simulink library "halin"  (R2021b)
settings: Solver=VariableStepAuto  StartTime=0.0  StopTime=10.0  RelTol=1e-3
undefined symbols (not defined in the file): KHAL_CAN1ABM1E2E_flg, KHAL_CAN1ESC1E2E_flg, KHAL_CAN1ESC5E2E_flg, KHAL_CAN1ESC7E2E_flg, KHAL_CAN1FCM2E2E_flg, KHAL_CAN1FCM3E2E_flg, KHAL_CAN1FCM4E2E_flg, KHAL_CAN3BMS1E2E_flg, KHAL_CAN3BMS6E2E_flg, KHAL_CAN3CCU1E2E_flg, KHAL_CAN3CCU2E2E_flg, KHAL_CAN3MCUF1E2E_flg, KHAL_CAN3MCUR1E2E_flg, KHAL_CAN3Shifter1E2E_flg, TRUE
libraries: simulink x420, FVT_lib x149, hcu_lib x49
(part 6 of 14)

== system halin/HAL_IN/CAN1/FCM3 ==
  DT_CAN1_SG_FCM3 : Inport
  0x82 : Constant  Value=0x82
  0xa0 : Constant  Value=0xa0
  ACCObjDist : Subsystem
  ACCObjRelSpd : Subsystem
  ADASForceIdle : Subsystem
  BitwiseAND{,1..9} (10 alike) : simulink/Logic and Bit Operations/Bitwise Operator  logicop=AND  UseBitMask=on  BitMask=0xFF  BitMaskRealWorld=Stored Integer
  BitwiseOR{,2,4..5} (4 alike) : simulink/Logic and Bit Operations/Bitwise Operator  logicop=OR  UseBitMask=off  BitMask=bin2dec('11011001')  BitMaskRealWorld=Stored Integer
  BitwiseOR1 : simulink/Logic and Bit Operations/Bitwise Operator  logicop=OR  UseBitMask=off  NumInputPorts=3  BitMask=bin2dec('11011001')  BitMaskRealWorld=Stored Integer
  BitwiseOR3 : simulink/Logic and Bit Operations/Bitwise Operator  logicop=OR  UseBitMask=off  NumInputPorts=3  BitMask=bin2dec('11011001')  BitMaskRealWorld=Stored Integer
  DDM_CS&RC_Comparison : FVT_lib/hal/DDM_CS&RC_Comparison  MsgCycleTime=10
  Data Type Conversion{,1..9} (10 alike) : DataTypeConversion  OutDataTypeStr=uint8
  FCM3Checksum : Subsystem
  FCM3LifeCount : Subsystem
  KHAL_CAN1FCM3E2E_flg : Constant  Value=KHAL_CAN1FCM3E2E_flg
  LeftShift : ArithShift  BitShiftNumber=3  BitShiftDirection=Left
  LeftShift1 : ArithShift  BitShiftNumber=3  BitShiftDirection=Left
  LeftShift2 : ArithShift  BitShiftNumber=6  BitShiftDirection=Left
  LeftShift3 : ArithShift  BitShiftDirection=Left
  LeftShift4 : ArithShift  BitShiftDirection=Left
  LeftShift5 : ArithShift  BitShiftNumber=4  BitShiftDirection=Left
  MessageRollingCounter : FVT_lib/hal/MessageRollingCounter  CounterMAX=14  task_time_ms=5  msg_time_ms=10
  Mux : Mux  Inputs=7
  RightShift : ArithShift  BitShiftNumber=8
  RightShift1 : ArithShift
  RightShift2 : ArithShift  BitShiftNumber=8
  RightShift3 : ArithShift
  bus_selector : BusSelector  OutputSignals=CAN1_ACC_ObjDist,CAN1_ACC_ObjRelSpd,CAN1_ADAS_ForceIdle,CAN1_ADAS_ShftPosnReq,CAN1_ADAS_ShftPosnReq_A,CAN1_ADAS_VehSpdLim,CAN1_FCM3_Checksum,CAN1_FCM3_LifeCount
  bus_selector1 : BusSelector  OutputSignals=CAN1_ACC_ObjDist
  bus_selector2 : BusSelector  OutputSignals=CAN1_ACC_ObjRelSpd
  bus_selector3 : BusSelector  OutputSignals=CAN1_ADAS_ForceIdle
  bus_selector4 : BusSelector  OutputSignals=CAN1_FCM3_Checksum
  bus_selector5 : BusSelector  OutputSignals=CAN1_FCM3_LifeCount
  constant : Constant  Value=0x0  OutDataTypeStr=uint8
  constant1 : Constant  Value=0x0  OutDataTypeStr=uint8
  VHAL_FCM3CSErr_flg : Outport
  VHAL_FCM3RCErr_flg : Outport  Port=2
  VHAL_ACCObjDist_m : Outport  Port=3
  VHAL_ACCObjRelSpd_mps : Outport  Port=4
  VHAL_ADASForceIdle_flg : Outport  Port=5
  VHAL_FCM3Checksum_enum : Outport  Port=6
  VHAL_FCM3LifeCount_enum : Outport  Port=7
  wires:
  DT_CAN1_SG_FCM3/1 -> [DT_CAN1_SG_FCM3]
  [DT_CAN1_SG_FCM3] -> bus_selector/1
  bus_selector/1 -> [CAN1_ACC_ObjDist]  "<CAN1_ACC_ObjDist>"
  [CAN1_ACC_ObjDist] -> RightShift/1, RightShift1/1
  RightShift/1 -> BitwiseAND/1
  BitwiseAND/1 -> [Byte_3_CAN1_ACC_ObjDist]
  RightShift1/1 -> BitwiseAND1/1
  BitwiseAND1/1 -> [Byte_4_CAN1_ACC_ObjDist]
  bus_selector/2 -> [CAN1_ACC_ObjRelSpd]  "<CAN1_ACC_ObjRelSpd>"
  [CAN1_ACC_ObjRelSpd] -> RightShift2/1, RightShift3/1
  RightShift2/1 -> BitwiseAND2/1
  BitwiseAND2/1 -> [Byte_5_CAN1_ACC_ObjRelSpd]
  RightShift3/1 -> BitwiseAND3/1
  BitwiseAND3/1 -> [Byte_6_CAN1_ACC_ObjRelSpd]
  bus_selector/3 -> [CAN1_ADAS_ForceIdle]  "<CAN1_ADAS_ForceIdle>"
  [CAN1_ADAS_ForceIdle] -> LeftShift/1
  LeftShift/1 -> BitwiseAND4/1
  BitwiseAND4/1 -> [Byte_5_CAN1_ADAS_ForceIdle]
  bus_selector/4 -> [CAN1_ADAS_ShftPosnReq]  "<CAN1_ADAS_ShftPosnReq>"
  [CAN1_ADAS_ShftPosnReq] -> LeftShift1/1
  LeftShift1/1 -> BitwiseAND5/1
  BitwiseAND5/1 -> [Byte_3_CAN1_ADAS_ShftPosnReq]
  bus_selector/5 -> [CAN1_ADAS_ShftPosnReq_A]  "<CAN1_ADAS_ShftPosnReq_A>"
  [CAN1_ADAS_ShftPosnReq_A] -> LeftShift2/1
  LeftShift2/1 -> BitwiseAND6/1
  BitwiseAND6/1 -> [Byte_3_CAN1_ADAS_ShftPosnReq_A]
  bus_selector/6 -> [CAN1_ADAS_VehSpdLim]  "<CAN1_ADAS_VehSpdLim>"
  [CAN1_ADAS_VehSpdLim] -> LeftShift3/1
  LeftShift3/1 -> BitwiseAND7/1
  BitwiseAND7/1 -> [Byte_0_CAN1_ADAS_VehSpdLim]
  bus_selector/7 -> [CAN1_FCM3_Checksum]  "<CAN1_FCM3_Checksum>"
  [CAN1_FCM3_Checksum] -> LeftShift4/1
  LeftShift4/1 -> BitwiseAND8/1
  BitwiseAND8/1 -> [Byte_7_CAN1_FCM3_Checksum]
  bus_selector/8 -> [CAN1_FCM3_LifeCount]  "<CAN1_FCM3_LifeCount>"
  [CAN1_FCM3_LifeCount] -> LeftShift5/1
  LeftShift5/1 -> BitwiseAND9/1
  BitwiseAND9/1 -> [Byte_5_CAN1_FCM3_LifeCount]
  Data Type Conversion/1 -> BitwiseOR/1
  [Byte_0_CAN1_ADAS_VehSpdLim] -> Data Type Conversion/1
  BitwiseOR/1 -> [Byte_0]
  constant/1 -> [Byte_1]
  constant1/1 -> [Byte_2]
  Data Type Conversion1/1 -> BitwiseOR1/1
  [Byte_3_CAN1_ACC_ObjDist] -> Data Type Conversion1/1
  Data Type Conversion2/1 -> BitwiseOR1/2
  [Byte_3_CAN1_ADAS_ShftPosnReq] -> Data Type Conversion2/1
  Data Type Conversion3/1 -> BitwiseOR1/3
  [Byte_3_CAN1_ADAS_ShftPosnReq_A] -> Data Type Conversion3/1
  BitwiseOR1/1 -> [Byte_3]
  Data Type Conversion4/1 -> BitwiseOR2/1
  [Byte_4_CAN1_ACC_ObjDist] -> Data Type Conversion4/1
  BitwiseOR2/1 -> [Byte_4]
  Data Type Conversion5/1 -> BitwiseOR3/1
  [Byte_5_CAN1_ACC_ObjRelSpd] -> Data Type Conversion5/1
  Data Type Conversion6/1 -> BitwiseOR3/2
  [Byte_5_CAN1_ADAS_ForceIdle] -> Data Type Conversion6/1
  Data Type Conversion7/1 -> BitwiseOR3/3
  [Byte_5_CAN1_FCM3_LifeCount] -> Data Type Conversion7/1
  BitwiseOR3/1 -> [Byte_5]
  Data Type Conversion8/1 -> BitwiseOR4/1
  [Byte_6_CAN1_ACC_ObjRelSpd] -> Data Type Conversion8/1
  BitwiseOR4/1 -> [Byte_6]
  Data Type Conversion9/1 -> BitwiseOR5/1
  [Byte_7_CAN1_FCM3_Checksum] -> Data Type Conversion9/1
  BitwiseOR5/1 -> [Byte_7]
  [Byte_0] -> Mux/1
  [Byte_1] -> Mux/2
  [Byte_2] -> Mux/3
  [Byte_3] -> Mux/4
  [Byte_4] -> Mux/5
  [Byte_5] -> Mux/6
  [Byte_6] -> Mux/7
  Mux/1 -> [VHAL_CAN1FCM3noCS_raw]
  KHAL_CAN1FCM3E2E_flg/1 -> DDM_CS&RC_Comparison/1
  0xa0/1 -> DDM_CS&RC_Comparison/2
  0x82/1 -> DDM_CS&RC_Comparison/3
  [VHAL_CAN1FCM3noCS_raw] -> DDM_CS&RC_Comparison/4
  [Byte_7] -> DDM_CS&RC_Comparison/5
  [RC_ECU] -> DDM_CS&RC_Comparison/6
  MessageRollingCounter/1 -> DDM_CS&RC_Comparison/7
  DDM_CS&RC_Comparison/1 -> VHAL_FCM3CSErr_flg/1
  DDM_CS&RC_Comparison/2 -> VHAL_FCM3RCErr_flg/1
  [DT_CAN1_SG_FCM3] -> bus_selector1/1
  bus_selector1/1 -> ACCObjDist/1(ACC_ObjDist)  "<CAN1_ACC_ObjDist>"
  ACCObjDist/1(VHAL_ACCObjDist_m) -> VHAL_ACCObjDist_m/1
  [DT_CAN1_SG_FCM3] -> bus_selector2/1
  bus_selector2/1 -> ACCObjRelSpd/1(ACC_ObjRelSpd)  "<CAN1_ACC_ObjRelSpd>"
  ACCObjRelSpd/1(VHAL_ACCObjRelSpd_mps) -> VHAL_ACCObjRelSpd_mps/1
  [DT_CAN1_SG_FCM3] -> bus_selector3/1
  bus_selector3/1 -> ADASForceIdle/1(ADAS_ForceIdle)  "<CAN1_ADAS_ForceIdle>"
  ADASForceIdle/1(VHAL_ADASForceIdle_flg) -> VHAL_ADASForceIdle_flg/1
  [DT_CAN1_SG_FCM3] -> bus_selector4/1
  bus_selector4/1 -> FCM3Checksum/1(FCM3_Checksum)  "<CAN1_FCM3_Checksum>"
  FCM3Checksum/1(VHAL_FCM3Checksum_enum) -> VHAL_FCM3Checksum_enum/1
  [DT_CAN1_SG_FCM3] -> bus_selector5/1
  bus_selector5/1 -> FCM3LifeCount/1(FCM3_LifeCount)  "<CAN1_FCM3_LifeCount>"
  FCM3LifeCount/1(VHAL_FCM3LifeCount_enum) -> VHAL_FCM3LifeCount_enum/1, [RC_ECU]

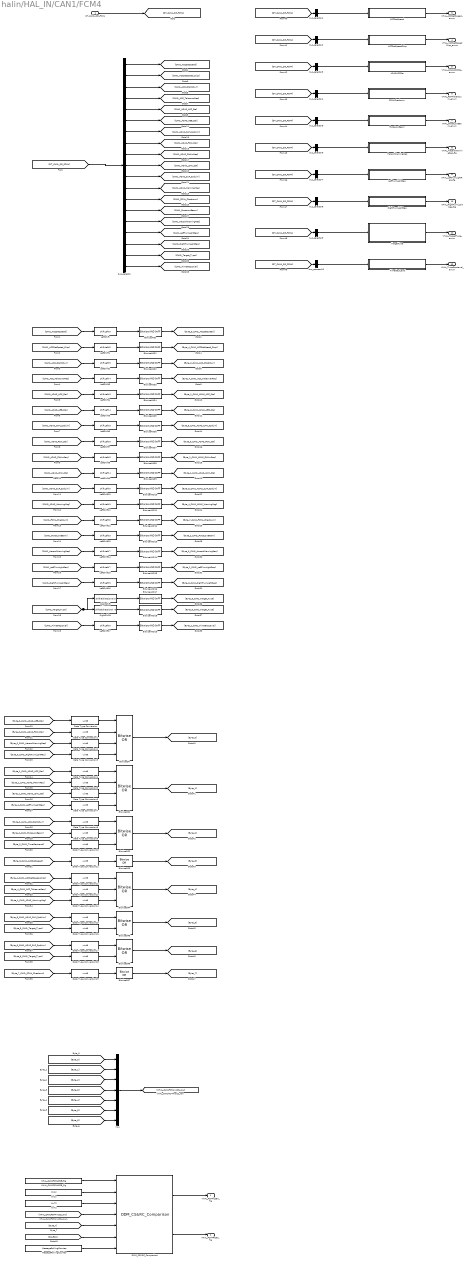
== system halin/HAL_IN/CAN1/FCM4 ==
  DT_CAN1_SG_FCM4 : Inport
  0x1c : Constant  Value=0x1c
  0x72 : Constant  Value=0x72
  ACCSetSpeed : Subsystem
  ACCSetSpeedDisp : Subsystem
  ADASACCSta : Subsystem
  BitwiseAND{,1..19} (20 alike) : simulink/Logic and Bit Operations/Bitwise Operator  logicop=AND  UseBitMask=on  BitMask=0xFF  BitMaskRealWorld=Stored Integer
  BitwiseOR : simulink/Logic and Bit Operations/Bitwise Operator  logicop=OR  UseBitMask=off  NumInputPorts=4  BitMask=bin2dec('11011001')  BitMaskRealWorld=Stored Integer
  BitwiseOR1 : simulink/Logic and Bit Operations/Bitwise Operator  logicop=OR  UseBitMask=off  NumInputPorts=4  BitMask=bin2dec('11011001')  BitMaskRealWorld=Stored Integer
  BitwiseOR2 : simulink/Logic and Bit Operations/Bitwise Operator  logicop=OR  UseBitMask=off  NumInputPorts=3  BitMask=bin2dec('11011001')  BitMaskRealWorld=Stored Integer
  BitwiseOR3 : simulink/Logic and Bit Operations/Bitwise Operator  logicop=OR  UseBitMask=off  BitMask=bin2dec('11011001')  BitMaskRealWorld=Stored Integer
  BitwiseOR4 : simulink/Logic and Bit Operations/Bitwise Operator  logicop=OR  UseBitMask=off  NumInputPorts=3  BitMask=bin2dec('11011001')  BitMaskRealWorld=Stored Integer
  BitwiseOR5 : simulink/Logic and Bit Operations/Bitwise Operator  logicop=OR  UseBitMask=off  NumInputPorts=2  BitMask=bin2dec('11011001')  BitMaskRealWorld=Stored Integer
  BitwiseOR6 : simulink/Logic and Bit Operations/Bitwise Operator  logicop=OR  UseBitMask=off  NumInputPorts=2  BitMask=bin2dec('11011001')  BitMaskRealWorld=Stored Integer
  BitwiseOR7 : simulink/Logic and Bit Operations/Bitwise Operator  logicop=OR  UseBitMask=off  BitMask=bin2dec('11011001')  BitMaskRealWorld=Stored Integer
  DDM_CS&RC_Comparison : FVT_lib/hal/DDM_CS&RC_Comparison  MsgCycleTime=100
  Data Type Conversion{,1..19} (20 alike) : DataTypeConversion  OutDataTypeStr=uint8
  FCM4Checksum : Subsystem
  ForceLowBeam : Subsystem
  HazardWarningReq : Subsystem
  KHAL_CAN1FCM4E2E_flg : Constant  Value=KHAL_CAN1FCM4E2E_flg
  LeftShift{,4,7,10..12,17} (7 alike) : ArithShift  BitShiftDirection=Left
  LeftShift1 : ArithShift  BitShiftNumber=5  BitShiftDirection=Left
  LeftShift{6,8,13,16} (4 alike) : ArithShift  BitShiftNumber=3  BitShiftDirection=Left
  LeftShift14 : ArithShift  BitShiftNumber=7  BitShiftDirection=Left
  LeftShift15 : ArithShift  BitShiftNumber=7  BitShiftDirection=Left
  LeftShift2 : ArithShift  BitShiftNumber=5  BitShiftDirection=Left
  LeftShift3 : ArithShift  BitShiftNumber=4  BitShiftDirection=Left
  LeftShift5 : ArithShift  BitShiftNumber=4  BitShiftDirection=Left
  LeftShift9 : ArithShift  BitShiftNumber=4  BitShiftDirection=Left
  LeftTurnLightReq : Subsystem
  MessageRollingCounter : FVT_lib/hal/MessageRollingCounter  CounterMAX=14  task_time_ms=5  msg_time_ms=100
  Mux : Mux  Inputs=7
  RightShift : ArithShift  BitShiftNumber=3
  RightShift1 : ArithShift  BitShiftNumber=-5
  RightTurnLightReq : Subsystem
  TargetType : Subsystem
  TimeGapLevel : Subsystem
  bus_selector : BusSelector  OutputSignals=CAN1_ACCSetSpeed,CAN1_ACCSetSpeed_Disp,CAN1_ACC_ObjDstLvl,CAN1_ACC_TakeoverReq,CAN1_ADAS_ACC_Sta,CAN1_ADAS_AEB_Sta,CAN1_ADAS_CAM_SpdLim,CAN1_ADAS_FCW_Sta,CAN1_ADAS_FltWrnReq,CAN1_ADAS_LDW_Sta,CAN1_ADAS_SLIF_SpdLim,CAN1_ADAS_WarningMsg,CAN1_FCM4_Checksum,CAN1_ForceLowBeam,CAN1_HazardWarningReq,CAN1_LeftTurnLightReq,CAN1_RightTurnLightReq,CAN1_Target_Type,CAN1_TimeGapLevel
  bus_selector1 : BusSelector  OutputSignals=CAN1_ACCSetSpeed
  bus_selector10 : BusSelector  OutputSignals=CAN1_TimeGapLevel
  bus_selector2 : BusSelector  OutputSignals=CAN1_ACCSetSpeed_Disp
  bus_selector3 : BusSelector  OutputSignals=CAN1_ADAS_ACC_Sta
  bus_selector4 : BusSelector  OutputSignals=CAN1_FCM4_Checksum
  bus_selector5 : BusSelector  OutputSignals=CAN1_ForceLowBeam
  bus_selector6 : BusSelector  OutputSignals=CAN1_HazardWarningReq
  bus_selector7 : BusSelector  OutputSignals=CAN1_LeftTurnLightReq
  bus_selector8 : BusSelector  OutputSignals=CAN1_RightTurnLightReq
  bus_selector9 : BusSelector  OutputSignals=CAN1_Target_Type
  VHAL_FCM4CSErr_flg : Outport
  VHAL_FCM4RCErr_flg : Outport  Port=2
  VHAL_ACCSetSpeed_enum : Outport  Port=3
  VHAL_ACCSetSpeedDisp_enum : Outport  Port=4
  VHAL_ADASACCSta_enum : Outport  Port=5
  VHAL_FCM4Checksum_enum : Outport  Port=6
  VHAL_ForceLowBeam_enum : Outport  Port=7
  VHAL_HazardWarningReq_flg : Outport  Port=8
  VHAL_LeftTurnLightReq_flg : Outport  Port=9
  VHAL_RightTurnLightReq_flg : Outport  Port=10
  VHAL_TargetType_enum : Outport  Port=11
  VHAL_TimeGapLevel_enum : Outport  Port=12
  wires:
  DT_CAN1_SG_FCM4/1 -> [DT_CAN1_SG_FCM4]
  [DT_CAN1_SG_FCM4] -> bus_selector/1
  bus_selector/1 -> [CAN1_ACCSetSpeed]  "<CAN1_ACCSetSpeed>"
  [CAN1_ACCSetSpeed] -> LeftShift/1
  LeftShift/1 -> BitwiseAND/1
  BitwiseAND/1 -> [Byte_3_CAN1_ACCSetSpeed]
  bus_selector/2 -> [CAN1_ACCSetSpeed_Disp]  "<CAN1_ACCSetSpeed_Disp>"
  [CAN1_ACCSetSpeed_Disp] -> LeftShift1/1
  LeftShift1/1 -> BitwiseAND1/1
  BitwiseAND1/1 -> [Byte_4_CAN1_ACCSetSpeed_Disp]
  bus_selector/3 -> [CAN1_ACC_ObjDstLvl]  "<CAN1_ACC_ObjDstLvl>"
  [CAN1_ACC_ObjDstLvl] -> LeftShift2/1
  LeftShift2/1 -> BitwiseAND2/1
  BitwiseAND2/1 -> [Byte_2_CAN1_ACC_ObjDstLvl]
  bus_selector/4 -> [CAN1_ACC_TakeoverReq]  "<CAN1_ACC_TakeoverReq>"
  [CAN1_ACC_TakeoverReq] -> LeftShift3/1
  LeftShift3/1 -> BitwiseAND3/1
  BitwiseAND3/1 -> [Byte_4_CAN1_ACC_TakeoverReq]
  bus_selector/5 -> [CAN1_ADAS_ACC_Sta]  "<CAN1_ADAS_ACC_Sta>"
  [CAN1_ADAS_ACC_Sta] -> LeftShift4/1
  LeftShift4/1 -> BitwiseAND4/1
  BitwiseAND4/1 -> [Byte_1_CAN1_ADAS_ACC_Sta]
  bus_selector/6 -> [CAN1_ADAS_AEB_Sta]  "<CAN1_ADAS_AEB_Sta>"
  [CAN1_ADAS_AEB_Sta] -> LeftShift5/1
  LeftShift5/1 -> BitwiseAND5/1
  BitwiseAND5/1 -> [Byte_0_CAN1_ADAS_AEB_Sta]
  bus_selector/7 -> [CAN1_ADAS_CAM_SpdLim]  "<CAN1_ADAS_CAM_SpdLim>"
  [CAN1_ADAS_CAM_SpdLim] -> LeftShift6/1
  LeftShift6/1 -> BitwiseAND6/1
  BitwiseAND6/1 -> [Byte_5_CAN1_ADAS_CAM_SpdLim]
  bus_selector/8 -> [CAN1_ADAS_FCW_Sta]  "<CAN1_ADAS_FCW_Sta>"
  [CAN1_ADAS_FCW_Sta] -> LeftShift7/1
  LeftShift7/1 -> BitwiseAND7/1
  BitwiseAND7/1 -> [Byte_0_CAN1_ADAS_FCW_Sta]
  bus_selector/9 -> [CAN1_ADAS_FltWrnReq]  "<CAN1_ADAS_FltWrnReq>"
  [CAN1_ADAS_FltWrnReq] -> LeftShift8/1
  LeftShift8/1 -> BitwiseAND8/1
  BitwiseAND8/1 -> [Byte_1_CAN1_ADAS_FltWrnReq]
  bus_selector/10 -> [CAN1_ADAS_LDW_Sta]  "<CAN1_ADAS_LDW_Sta>"
  [CAN1_ADAS_LDW_Sta] -> LeftShift9/1
  LeftShift9/1 -> BitwiseAND9/1
  BitwiseAND9/1 -> [Byte_1_CAN1_ADAS_LDW_Sta]
  bus_selector/11 -> [CAN1_ADAS_SLIF_SpdLim]  "<CAN1_ADAS_SLIF_SpdLim>"
  [CAN1_ADAS_SLIF_SpdLim] -> LeftShift10/1
  LeftShift10/1 -> BitwiseAND10/1
  BitwiseAND10/1 -> [Byte_6_CAN1_ADAS_SLIF_SpdLim]
  bus_selector/12 -> [CAN1_ADAS_WarningMsg]  "<CAN1_ADAS_WarningMsg>"
  [CAN1_ADAS_WarningMsg] -> LeftShift11/1
  LeftShift11/1 -> BitwiseAND11/1
  BitwiseAND11/1 -> [Byte_4_CAN1_ADAS_WarningMsg]
  bus_selector/13 -> [CAN1_FCM4_Checksum]  "<CAN1_FCM4_Checksum>"
  [CAN1_FCM4_Checksum] -> LeftShift12/1
  LeftShift12/1 -> BitwiseAND12/1
  BitwiseAND12/1 -> [Byte_7_CAN1_FCM4_Checksum]
  bus_selector/14 -> [CAN1_ForceLowBeam]  "<CAN1_ForceLowBeam>"
  [CAN1_ForceLowBeam] -> LeftShift13/1
  LeftShift13/1 -> BitwiseAND13/1
  BitwiseAND13/1 -> [Byte_2_CAN1_ForceLowBeam]
  bus_selector/15 -> [CAN1_HazardWarningReq]  "<CAN1_HazardWarningReq>"
  [CAN1_HazardWarningReq] -> LeftShift14/1
  LeftShift14/1 -> BitwiseAND14/1
  BitwiseAND14/1 -> [Byte_0_CAN1_HazardWarningReq]
  bus_selector/16 -> [CAN1_LeftTurnLightReq]  "<CAN1_LeftTurnLightReq>"
  [CAN1_LeftTurnLightReq] -> LeftShift15/1
  LeftShift15/1 -> BitwiseAND15/1
  BitwiseAND15/1 -> [Byte_1_CAN1_LeftTurnLightReq]
  bus_selector/17 -> [CAN1_RightTurnLightReq]  "<CAN1_RightTurnLightReq>"
  [CAN1_RightTurnLightReq] -> LeftShift16/1
  LeftShift16/1 -> BitwiseAND16/1
  BitwiseAND16/1 -> [Byte_0_CAN1_RightTurnLightReq]
  bus_selector/18 -> [CAN1_Target_Type]  "<CAN1_Target_Type>"
  [CAN1_Target_Type] -> RightShift/1, RightShift1/1
  RightShift/1 -> BitwiseAND17/1
  BitwiseAND17/1 -> [Byte_5_CAN1_Target_Type]
  RightShift1/1 -> BitwiseAND18/1
  BitwiseAND18/1 -> [Byte_6_CAN1_Target_Type]
  bus_selector/19 -> [CAN1_TimeGapLevel]  "<CAN1_TimeGapLevel>"
  [CAN1_TimeGapLevel] -> LeftShift17/1
  LeftShift17/1 -> BitwiseAND19/1
  BitwiseAND19/1 -> [Byte_2_CAN1_TimeGapLevel]
  Data Type Conversion/1 -> BitwiseOR/1
  [Byte_0_CAN1_ADAS_AEB_Sta] -> Data Type Conversion/1
  Data Type Conversion1/1 -> BitwiseOR/2
  [Byte_0_CAN1_ADAS_FCW_Sta] -> Data Type Conversion1/1
  Data Type Conversion2/1 -> BitwiseOR/3
  [Byte_0_CAN1_HazardWarningReq] -> Data Type Conversion2/1
  Data Type Conversion3/1 -> BitwiseOR/4
  [Byte_0_CAN1_RightTurnLightReq] -> Data Type Conversion3/1
  BitwiseOR/1 -> [Byte_0]
  Data Type Conversion4/1 -> BitwiseOR1/1
  [Byte_1_CAN1_ADAS_ACC_Sta] -> Data Type Conversion4/1
  Data Type Conversion5/1 -> BitwiseOR1/2
  [Byte_1_CAN1_ADAS_FltWrnReq] -> Data Type Conversion5/1
  Data Type Conversion6/1 -> BitwiseOR1/3
  [Byte_1_CAN1_ADAS_LDW_Sta] -> Data Type Conversion6/1
  Data Type Conversion7/1 -> BitwiseOR1/4
  [Byte_1_CAN1_LeftTurnLightReq] -> Data Type Conversion7/1
  BitwiseOR1/1 -> [Byte_1]
  Data Type Conversion8/1 -> BitwiseOR2/1
  [Byte_2_CAN1_ACC_ObjDstLvl] -> Data Type Conversion8/1
  Data Type Conversion9/1 -> BitwiseOR2/2
  [Byte_2_CAN1_ForceLowBeam] -> Data Type Conversion9/1
  Data Type Conversion10/1 -> BitwiseOR2/3
  [Byte_2_CAN1_TimeGapLevel] -> Data Type Conversion10/1
  BitwiseOR2/1 -> [Byte_2]
  Data Type Conversion11/1 -> BitwiseOR3/1
  [Byte_3_CAN1_ACCSetSpeed] -> Data Type Conversion11/1
  BitwiseOR3/1 -> [Byte_3]
  Data Type Conversion12/1 -> BitwiseOR4/1
  [Byte_4_CAN1_ACCSetSpeed_Disp] -> Data Type Conversion12/1
  Data Type Conversion13/1 -> BitwiseOR4/2
  [Byte_4_CAN1_ACC_TakeoverReq] -> Data Type Conversion13/1
  Data Type Conversion14/1 -> BitwiseOR4/3
  [Byte_4_CAN1_ADAS_WarningMsg] -> Data Type Conversion14/1
  BitwiseOR4/1 -> [Byte_4]
  Data Type Conversion15/1 -> BitwiseOR5/1
  [Byte_5_CAN1_ADAS_CAM_SpdLim] -> Data Type Conversion15/1
  Data Type Conversion16/1 -> BitwiseOR5/2
  [Byte_5_CAN1_Target_Type] -> Data Type Conversion16/1
  BitwiseOR5/1 -> [Byte_5]
  Data Type Conversion17/1 -> BitwiseOR6/1
  [Byte_6_CAN1_ADAS_SLIF_SpdLim] -> Data Type Conversion17/1
  Data Type Conversion18/1 -> BitwiseOR6/2
  [Byte_6_CAN1_Target_Type] -> Data Type Conversion18/1
  BitwiseOR6/1 -> [Byte_6]
  Data Type Conversion19/1 -> BitwiseOR7/1
  [Byte_7_CAN1_FCM4_Checksum] -> Data Type Conversion19/1
  BitwiseOR7/1 -> [Byte_7]
  [Byte_0] -> Mux/1
  [Byte_1] -> Mux/2
  [Byte_2] -> Mux/3
  [Byte_3] -> Mux/4
  [Byte_4] -> Mux/5
  [Byte_5] -> Mux/6
  [Byte_6] -> Mux/7
  Mux/1 -> [VHAL_CAN1FCM4noCS_raw]
  KHAL_CAN1FCM4E2E_flg/1 -> DDM_CS&RC_Comparison/1
  0x1c/1 -> DDM_CS&RC_Comparison/2
  0x72/1 -> DDM_CS&RC_Comparison/3
  [VHAL_CAN1FCM4noCS_raw] -> DDM_CS&RC_Comparison/4
  [Byte_7] -> DDM_CS&RC_Comparison/5
  [RC_ECU] -> DDM_CS&RC_Comparison/6
  MessageRollingCounter/1 -> DDM_CS&RC_Comparison/7
  DDM_CS&RC_Comparison/1 -> VHAL_FCM4CSErr_flg/1
  DDM_CS&RC_Comparison/2 -> VHAL_FCM4RCErr_flg/1
  [DT_CAN1_SG_FCM4] -> bus_selector1/1
  bus_selector1/1 -> ACCSetSpeed/1(ACCSetSpeed)  "<CAN1_ACCSetSpeed>"
  ACCSetSpeed/1(VHAL_ACCSetSpeed_enum) -> VHAL_ACCSetSpeed_enum/1
  [DT_CAN1_SG_FCM4] -> bus_selector2/1
  bus_selector2/1 -> ACCSetSpeedDisp/1(ACCSetSpeed_Disp)  "<CAN1_ACCSetSpeed_Disp>"
  ACCSetSpeedDisp/1(VHAL_ACCSetSpeedDisp_enum) -> VHAL_ACCSetSpeedDisp_enum/1
  [DT_CAN1_SG_FCM4] -> bus_selector3/1
  bus_selector3/1 -> ADASACCSta/1(ADAS_ACC_Sta)  "<CAN1_ADAS_ACC_Sta>"
  ADASACCSta/1(VHAL_ADASACCSta_enum) -> VHAL_ADASACCSta_enum/1
  [DT_CAN1_SG_FCM4] -> bus_selector4/1
  bus_selector4/1 -> FCM4Checksum/1(FCM4_Checksum)  "<CAN1_FCM4_Checksum>"
  FCM4Checksum/1(VHAL_FCM4Checksum_enum) -> VHAL_FCM4Checksum_enum/1
  [DT_CAN1_SG_FCM4] -> bus_selector5/1
  bus_selector5/1 -> ForceLowBeam/1(ForceLowBeam)  "<CAN1_ForceLowBeam>"
  ForceLowBeam/1(VHAL_ForceLowBeam_enum) -> VHAL_ForceLowBeam_enum/1
  [DT_CAN1_SG_FCM4] -> bus_selector6/1
  bus_selector6/1 -> HazardWarningReq/1(HazardWarningReq)  "<CAN1_HazardWarningReq>"
  HazardWarningReq/1(VHAL_HazardWarningReq_flg) -> VHAL_HazardWarningReq_flg/1
  [DT_CAN1_SG_FCM4] -> bus_selector7/1
  bus_selector7/1 -> LeftTurnLightReq/1(LeftTurnLightReq)  "<CAN1_LeftTurnLightReq>"
  LeftTurnLightReq/1(VHAL_LeftTurnLightReq_flg) -> VHAL_LeftTurnLightReq_flg/1
  [DT_CAN1_SG_FCM4] -> bus_selector8/1
  bus_selector8/1 -> RightTurnLightReq/1(RightTurnLightReq)  "<CAN1_RightTurnLightReq>"
  RightTurnLightReq/1(VHAL_RightTurnLightReq_flg) -> VHAL_RightTurnLightReq_flg/1
  [DT_CAN1_SG_FCM4] -> bus_selector9/1
  bus_selector9/1 -> TargetType/1(Target_Type)  "<CAN1_Target_Type>"
  TargetType/1(VHAL_TargetType_enum) -> VHAL_TargetType_enum/1
  [DT_CAN1_SG_FCM4] -> bus_selector10/1
  bus_selector10/1 -> TimeGapLevel/1(TimeGapLevel)  "<CAN1_TimeGapLevel>"
  TimeGapLevel/1(VHAL_TimeGapLevel_enum) -> VHAL_TimeGapLevel_enum/1

== system halin/HAL_IN/CAN1/SRR1 ==
  DT_CAN1_SG_SRR1 : Inport
  SRRBSDWarnL : Subsystem
  SRRBSDWarnR : Subsystem
  SRRODAWarnL : Subsystem
  SRRODAWarnR : Subsystem
  bus_selector : BusSelector  OutputSignals=CAN1_SRR_BSD_WarnL
  bus_selector1 : BusSelector  OutputSignals=CAN1_SRR_BSD_WarnR
  bus_selector2 : BusSelector  OutputSignals=CAN1_SRR_ODA_WarnL
  bus_selector3 : BusSelector  OutputSignals=CAN1_SRR_ODA_WarnR
  VHAL_SRRBSDWarnL_enum : Outport
  VHAL_SRRBSDWarnR_enum : Outport  Port=2
  VHAL_SRRODAWarnL_enum : Outport  Port=3
  VHAL_SRRODAWarnR_enum : Outport  Port=4
  wires:
  DT_CAN1_SG_SRR1/1 -> [DT_CAN1_SG_SRR1]
  [DT_CAN1_SG_SRR1] -> bus_selector/1
  bus_selector/1 -> SRRBSDWarnL/1(SRR_BSD_WarnL)  "<CAN1_SRR_BSD_WarnL>"
  SRRBSDWarnL/1(VHAL_SRRBSDWarnL_enum) -> VHAL_SRRBSDWarnL_enum/1
  [DT_CAN1_SG_SRR1] -> bus_selector1/1
  bus_selector1/1 -> SRRBSDWarnR/1(SRR_BSD_WarnR)  "<CAN1_SRR_BSD_WarnR>"
  SRRBSDWarnR/1(VHAL_SRRBSDWarnR_enum) -> VHAL_SRRBSDWarnR_enum/1
  [DT_CAN1_SG_SRR1] -> bus_selector2/1
  bus_selector2/1 -> SRRODAWarnL/1(SRR_ODA_WarnL)  "<CAN1_SRR_ODA_WarnL>"
  SRRODAWarnL/1(VHAL_SRRODAWarnL_enum) -> VHAL_SRRODAWarnL_enum/1
  [DT_CAN1_SG_SRR1] -> bus_selector3/1
  bus_selector3/1 -> SRRODAWarnR/1(SRR_ODA_WarnR)  "<CAN1_SRR_ODA_WarnR>"
  SRRODAWarnR/1(VHAL_SRRODAWarnR_enum) -> VHAL_SRRODAWarnR_enum/1

== system halin/HAL_IN/CAN1/VHAL_CANMsgInvalidABM1_flg ==
  Cast To Boolean13 : DataTypeConversion  OutDataTypeStr=boolean
  Constant : Constant  Value=TRUE
  Latch13 : hcu_lib/Basic_Blocks/Latch
  Switch13 : Switch  Criteria=u2 ~= 0
  Unit Delay : UnitDelay  SampleTime=-1  HasFrameUpgradeWarning=on
  UnitConverter : DataTypeConversion  OutDataTypeStr=boolean
  Out : Outport
  wires:
  Constant/1 -> Switch13/3
  Unit Delay/1 -> Cast To Boolean13/1
  Cast To Boolean13/1 -> Switch13/1, Latch13/1
  Switch13/1 -> UnitConverter/1
  Latch13/1 -> Switch13/2
  UnitConverter/1 -> Unit Delay/1, Out/1  "VHAL_CANMsgInvalidABM1_flg"

== system halin/HAL_IN/CAN1/VHAL_CANMsgInvalidEPAS1_flg ==
  Cast To Boolean13 : DataTypeConversion  OutDataTypeStr=boolean
  Constant : Constant  Value=TRUE
  Latch13 : hcu_lib/Basic_Blocks/Latch
  Switch13 : Switch  Criteria=u2 ~= 0
  Unit Delay : UnitDelay  SampleTime=-1  HasFrameUpgradeWarning=on
  UnitConverter : DataTypeConversion  OutDataTypeStr=boolean
  Out : Outport
  wires:
  Constant/1 -> Switch13/3
  Unit Delay/1 -> Cast To Boolean13/1
  Cast To Boolean13/1 -> Switch13/1, Latch13/1
  Switch13/1 -> UnitConverter/1
  Latch13/1 -> Switch13/2
  UnitConverter/1 -> Unit Delay/1, Out/1  "VHAL_CANMsgInvalidEPAS1_flg"

== system halin/HAL_IN/CAN1/VHAL_CANMsgInvalidEPAS2_flg ==
  Cast To Boolean13 : DataTypeConversion  OutDataTypeStr=boolean
  Constant : Constant  Value=TRUE
  Latch13 : hcu_lib/Basic_Blocks/Latch
  Switch13 : Switch  Criteria=u2 ~= 0
  Unit Delay : UnitDelay  SampleTime=-1  HasFrameUpgradeWarning=on
  UnitConverter : DataTypeConversion  OutDataTypeStr=boolean
  Out : Outport
  wires:
  Constant/1 -> Switch13/3
  Unit Delay/1 -> Cast To Boolean13/1
  Cast To Boolean13/1 -> Switch13/1, Latch13/1
  Switch13/1 -> UnitConverter/1
  Latch13/1 -> Switch13/2
  UnitConverter/1 -> Unit Delay/1, Out/1  "VHAL_CANMsgInvalidEPAS2_flg"

== system halin/HAL_IN/CAN1/VHAL_CANMsgInvalidEPB1_flg ==
  Cast To Boolean13 : DataTypeConversion  OutDataTypeStr=boolean
  Constant : Constant  Value=TRUE
  Latch13 : hcu_lib/Basic_Blocks/Latch
  Switch13 : Switch  Criteria=u2 ~= 0
  Unit Delay : UnitDelay  SampleTime=-1  HasFrameUpgradeWarning=on
  UnitConverter : DataTypeConversion  OutDataTypeStr=boolean
  Out : Outport
  wires:
  Constant/1 -> Switch13/3
  Unit Delay/1 -> Cast To Boolean13/1
  Cast To Boolean13/1 -> Switch13/1, Latch13/1
  Switch13/1 -> UnitConverter/1
  Latch13/1 -> Switch13/2
  UnitConverter/1 -> Unit Delay/1, Out/1  "VHAL_CANMsgInvalidEPB1_flg"

== system halin/HAL_IN/CAN1/VHAL_CANMsgInvalidESC1_flg ==
  Cast To Boolean13 : DataTypeConversion  OutDataTypeStr=boolean
  Constant : Constant  Value=TRUE
  Latch13 : hcu_lib/Basic_Blocks/Latch
  Switch13 : Switch  Criteria=u2 ~= 0
  Unit Delay : UnitDelay  SampleTime=-1  HasFrameUpgradeWarning=on
  UnitConverter : DataTypeConversion  OutDataTypeStr=boolean
  Out : Outport
  wires:
  Constant/1 -> Switch13/3
  Unit Delay/1 -> Cast To Boolean13/1
  Cast To Boolean13/1 -> Switch13/1, Latch13/1
  Switch13/1 -> UnitConverter/1
  Latch13/1 -> Switch13/2
  UnitConverter/1 -> Unit Delay/1, Out/1  "VHAL_CANMsgInvalidESC1_flg"

== system halin/HAL_IN/CAN1/VHAL_CANMsgInvalidESC2_flg ==
  Cast To Boolean13 : DataTypeConversion  OutDataTypeStr=boolean
  Constant : Constant  Value=TRUE
  Latch13 : hcu_lib/Basic_Blocks/Latch
  Switch13 : Switch  Criteria=u2 ~= 0
  Unit Delay : UnitDelay  SampleTime=-1  HasFrameUpgradeWarning=on
  UnitConverter : DataTypeConversion  OutDataTypeStr=boolean
  Out : Outport
  wires:
  Constant/1 -> Switch13/3
  Unit Delay/1 -> Cast To Boolean13/1
  Cast To Boolean13/1 -> Switch13/1, Latch13/1
  Switch13/1 -> UnitConverter/1
  Latch13/1 -> Switch13/2
  UnitConverter/1 -> Unit Delay/1, Out/1  "VHAL_CANMsgInvalidESC2_flg"

== system halin/HAL_IN/CAN1/VHAL_CANMsgInvalidESC3_flg ==
  Cast To Boolean13 : DataTypeConversion  OutDataTypeStr=boolean
  Constant : Constant  Value=TRUE
  Latch13 : hcu_lib/Basic_Blocks/Latch
  Switch13 : Switch  Criteria=u2 ~= 0
  Unit Delay : UnitDelay  SampleTime=-1  HasFrameUpgradeWarning=on
  UnitConverter : DataTypeConversion  OutDataTypeStr=boolean
  Out : Outport
  wires:
  Constant/1 -> Switch13/3
  Unit Delay/1 -> Cast To Boolean13/1
  Cast To Boolean13/1 -> Switch13/1, Latch13/1
  Switch13/1 -> UnitConverter/1
  Latch13/1 -> Switch13/2
  UnitConverter/1 -> Unit Delay/1, Out/1  "VHAL_CANMsgInvalidESC3_flg"

== system halin/HAL_IN/CAN1/VHAL_CANMsgInvalidESC4_flg ==
  Cast To Boolean13 : DataTypeConversion  OutDataTypeStr=boolean
  Constant : Constant  Value=TRUE
  Latch13 : hcu_lib/Basic_Blocks/Latch
  Switch13 : Switch  Criteria=u2 ~= 0
  Unit Delay : UnitDelay  SampleTime=-1  HasFrameUpgradeWarning=on
  UnitConverter : DataTypeConversion  OutDataTypeStr=boolean
  Out : Outport
  wires:
  Constant/1 -> Switch13/3
  Unit Delay/1 -> Cast To Boolean13/1
  Cast To Boolean13/1 -> Switch13/1, Latch13/1
  Switch13/1 -> UnitConverter/1
  Latch13/1 -> Switch13/2
  UnitConverter/1 -> Unit Delay/1, Out/1  "VHAL_CANMsgInvalidESC4_flg"

== system halin/HAL_IN/CAN1/VHAL_CANMsgInvalidESC5_flg ==
  Cast To Boolean13 : DataTypeConversion  OutDataTypeStr=boolean
  Constant : Constant  Value=TRUE
  Latch13 : hcu_lib/Basic_Blocks/Latch
  Switch13 : Switch  Criteria=u2 ~= 0
  Unit Delay : UnitDelay  SampleTime=-1  HasFrameUpgradeWarning=on
  UnitConverter : DataTypeConversion  OutDataTypeStr=boolean
  Out : Outport
  wires:
  Constant/1 -> Switch13/3
  Unit Delay/1 -> Cast To Boolean13/1
  Cast To Boolean13/1 -> Switch13/1, Latch13/1
  Switch13/1 -> UnitConverter/1
  Latch13/1 -> Switch13/2
  UnitConverter/1 -> Unit Delay/1, Out/1  "VHAL_CANMsgInvalidESC5_flg"

== system halin/HAL_IN/CAN1/VHAL_CANMsgInvalidESC6_flg ==
  Cast To Boolean13 : DataTypeConversion  OutDataTypeStr=boolean
  Constant : Constant  Value=TRUE
  Latch13 : hcu_lib/Basic_Blocks/Latch
  Switch13 : Switch  Criteria=u2 ~= 0
  Unit Delay : UnitDelay  SampleTime=-1  HasFrameUpgradeWarning=on
  UnitConverter : DataTypeConversion  OutDataTypeStr=boolean
  Out : Outport
  wires:
  Constant/1 -> Switch13/3
  Unit Delay/1 -> Cast To Boolean13/1
  Cast To Boolean13/1 -> Switch13/1, Latch13/1
  Switch13/1 -> UnitConverter/1
  Latch13/1 -> Switch13/2
  UnitConverter/1 -> Unit Delay/1, Out/1  "VHAL_CANMsgInvalidESC6_flg"

== system halin/HAL_IN/CAN1/VHAL_CANMsgInvalidESC7_flg ==
  Cast To Boolean13 : DataTypeConversion  OutDataTypeStr=boolean
  Constant : Constant  Value=TRUE
  Latch13 : hcu_lib/Basic_Blocks/Latch
  Switch13 : Switch  Criteria=u2 ~= 0
  Unit Delay : UnitDelay  SampleTime=-1  HasFrameUpgradeWarning=on
  UnitConverter : DataTypeConversion  OutDataTypeStr=boolean
  Out : Outport
  wires:
  Constant/1 -> Switch13/3
  Unit Delay/1 -> Cast To Boolean13/1
  Cast To Boolean13/1 -> Switch13/1, Latch13/1
  Switch13/1 -> UnitConverter/1
  Latch13/1 -> Switch13/2
  UnitConverter/1 -> Unit Delay/1, Out/1  "VHAL_CANMsgInvalidESC7_flg"

== system halin/HAL_IN/CAN1/VHAL_CANMsgInvalidFCM2_flg ==
  Cast To Boolean13 : DataTypeConversion  OutDataTypeStr=boolean
  Constant : Constant  Value=TRUE
  Latch13 : hcu_lib/Basic_Blocks/Latch
  Switch13 : Switch  Criteria=u2 ~= 0
  Unit Delay : UnitDelay  SampleTime=-1  HasFrameUpgradeWarning=on
  UnitConverter : DataTypeConversion  OutDataTypeStr=boolean
  Out : Outport
  wires:
  Constant/1 -> Switch13/3
  Unit Delay/1 -> Cast To Boolean13/1
  Cast To Boolean13/1 -> Switch13/1, Latch13/1
  Switch13/1 -> UnitConverter/1
  Latch13/1 -> Switch13/2
  UnitConverter/1 -> Unit Delay/1, Out/1  "VHAL_CANMsgInvalidFCM2_flg"

== system halin/HAL_IN/CAN1/VHAL_CANMsgInvalidFCM3_flg ==
  Cast To Boolean13 : DataTypeConversion  OutDataTypeStr=boolean
  Constant : Constant  Value=TRUE
  Latch13 : hcu_lib/Basic_Blocks/Latch
  Switch13 : Switch  Criteria=u2 ~= 0
  Unit Delay : UnitDelay  SampleTime=-1  HasFrameUpgradeWarning=on
  UnitConverter : DataTypeConversion  OutDataTypeStr=boolean
  Out : Outport
  wires:
  Constant/1 -> Switch13/3
  Unit Delay/1 -> Cast To Boolean13/1
  Cast To Boolean13/1 -> Switch13/1, Latch13/1
  Switch13/1 -> UnitConverter/1
  Latch13/1 -> Switch13/2
  UnitConverter/1 -> Unit Delay/1, Out/1  "VHAL_CANMsgInvalidFCM3_flg"

== system halin/HAL_IN/CAN1/VHAL_CANMsgInvalidFCM4_flg ==
  Cast To Boolean13 : DataTypeConversion  OutDataTypeStr=boolean
  Constant : Constant  Value=TRUE
  Latch13 : hcu_lib/Basic_Blocks/Latch
  Switch13 : Switch  Criteria=u2 ~= 0
  Unit Delay : UnitDelay  SampleTime=-1  HasFrameUpgradeWarning=on
  UnitConverter : DataTypeConversion  OutDataTypeStr=boolean
  Out : Outport
  wires:
  Constant/1 -> Switch13/3
  Unit Delay/1 -> Cast To Boolean13/1
  Cast To Boolean13/1 -> Switch13/1, Latch13/1
  Switch13/1 -> UnitConverter/1
  Latch13/1 -> Switch13/2
  UnitConverter/1 -> Unit Delay/1, Out/1  "VHAL_CANMsgInvalidFCM4_flg"

== system halin/HAL_IN/CAN1/VHAL_CANMsgInvalidSRR1_flg ==
  Cast To Boolean13 : DataTypeConversion  OutDataTypeStr=boolean
  Constant : Constant  Value=TRUE
  Latch13 : hcu_lib/Basic_Blocks/Latch
  Switch13 : Switch  Criteria=u2 ~= 0
  Unit Delay : UnitDelay  SampleTime=-1  HasFrameUpgradeWarning=on
  UnitConverter : DataTypeConversion  OutDataTypeStr=boolean
  Out : Outport
  wires:
  Constant/1 -> Switch13/3
  Unit Delay/1 -> Cast To Boolean13/1
  Cast To Boolean13/1 -> Switch13/1, Latch13/1
  Switch13/1 -> UnitConverter/1
  Latch13/1 -> Switch13/2
  UnitConverter/1 -> Unit Delay/1, Out/1  "VHAL_CANMsgInvalidSRR1_flg"

== system halin/HAL_IN/CAN2/IVI1 ==
  DT_CAN2_SG_IVI1 : Inport
  AmbLightColorSet : Subsystem
  AmbLightUserSet : Subsystem
  BrkAbnGoReadySW : Subsystem
  DRAmbLightBrightnessSet : Subsystem
  FCPFrEvtBtnACMaxReq : Subsystem
  FCPFrEvtBtnACReq : Subsystem
  FCPFrEvtBtnAutoReq : Subsystem
  FCPFrEvtBtnSyncReq : Subsystem
  FCPMidEvtBtnAutoReq : Subsystem
  IPAmbLightBrightnessSet : Subsystem
  IVILockSoundSWSta : Subsystem
  IVIOTAUpdSta : Subsystem
  LINKtoDrive : Subsystem
  OTACancelDLReq : Subsystem
  OTACompNTFYPres : Subsystem
  OTADLReq : Subsystem
  OTASuspendDLReq : Subsystem
  OTAUpdStartReq : Subsystem
  OpenDrOpenWdoSW : Subsystem
  PWCLOSEIMD : Subsystem
  PWCONTINUEUSE : Subsystem
  SchedOTAwake : Subsystem
  SmartEcoModeSW : Subsystem
  UpdCountdownCancel : Subsystem
  UpdCountdownSkip : Subsystem
  VehACModReq : Subsystem
  bus_selector : BusSelector  OutputSignals=CAN2_AmbLightColorSet
  bus_selector1 : BusSelector  OutputSignals=CAN2_AmbLightUserSet
  bus_selector10 : BusSelector  OutputSignals=CAN2_IVI_Lock_SoundSW_Sta
  bus_selector11 : BusSelector  OutputSignals=CAN2_IVI_OTA_Upd_Sta
  bus_selector12 : BusSelector  OutputSignals=CAN2_LINKtoDrive
  bus_selector13 : BusSelector  OutputSignals=CAN2_OTA_CancelDL_Req
  bus_selector14 : BusSelector  OutputSignals=CAN2_OTA_CompNTFY_Pres
  bus_selector15 : BusSelector  OutputSignals=CAN2_OTA_DL_Req
  bus_selector16 : BusSelector  OutputSignals=CAN2_OTA_SuspendDL_Req
  bus_selector17 : BusSelector  OutputSignals=CAN2_OTA_UpdStart_Req
  bus_selector18 : BusSelector  OutputSignals=CAN2_OpenDrOpenWdo_SW
  bus_selector19 : BusSelector  OutputSignals=CAN2_PW_CLOSE_IMD
  bus_selector2 : BusSelector  OutputSignals=CAN2_BrkAbn_GoReady_SW
  bus_selector20 : BusSelector  OutputSignals=CAN2_PW_CONTINUE_USE
  bus_selector21 : BusSelector  OutputSignals=CAN2_Sched_OTA_wake
  bus_selector22 : BusSelector  OutputSignals=CAN2_SmartEco_Mode_SW
  bus_selector23 : BusSelector  OutputSignals=CAN2_Upd_Countdown_Cancel
  bus_selector24 : BusSelector  OutputSignals=CAN2_Upd_Countdown_Skip
  bus_selector25 : BusSelector  OutputSignals=CAN2_VehACModReq
  bus_selector3 : BusSelector  OutputSignals=CAN2_DRAmbLightBrightnessSet
  bus_selector4 : BusSelector  OutputSignals=CAN2_FCP_FrEvt_BtnACMaxReq
  bus_selector5 : BusSelector  OutputSignals=CAN2_FCP_FrEvt_BtnACReq
  bus_selector6 : BusSelector  OutputSignals=CAN2_FCP_FrEvt_BtnAutoReq
  bus_selector7 : BusSelector  OutputSignals=CAN2_FCP_FrEvt_BtnSyncReq
  bus_selector8 : BusSelector  OutputSignals=CAN2_FCP_MidEvt_BtnAutoReq
  bus_selector9 : BusSelector  OutputSignals=CAN2_IPAmbLightBrightnessSet
  VHAL_AmbLightColorSet_enum : Outport
  VHAL_AmbLightUserSet_enum : Outport  Port=2
  VHAL_BrkAbnGoReadySW_flg : Outport  Port=3
  VHAL_DRAmbLightBrightnessSet_pct : Outport  Port=4
  VHAL_FCPFrEvtBtnACMaxReq_flg : Outport  Port=5
  VHAL_FCPFrEvtBtnACReq_flg : Outport  Port=6
  VHAL_FCPFrEvtBtnAutoReq_flg : Outport  Port=7
  VHAL_FCPFrEvtBtnSyncReq_flg : Outport  Port=8
  VHAL_FCPMidEvtBtnAutoReq_flg : Outport  Port=9
  VHAL_IPAmbLightBrightnessSet_pct : Outport  Port=10
  VHAL_IVILockSoundSWSta_flg : Outport  Port=11
  VHAL_IVIOTAUpdSta_enum : Outport  Port=12
  VHAL_LINKtoDrive_flg : Outport  Port=13
  VHAL_OTACancelDLReq_flg : Outport  Port=14
  VHAL_OTACompNTFYPres_flg : Outport  Port=15
  VHAL_OTADLReq_flg : Outport  Port=16
  VHAL_OTASuspendDLReq_flg : Outport  Port=17
  VHAL_OTAUpdStartReq_flg : Outport  Port=18
  VHAL_OpenDrOpenWdoSW_flg : Outport  Port=19
  VHAL_PWCLOSEIMD_flg : Outport  Port=20
  VHAL_PWCONTINUEUSE_flg : Outport  Port=21
  VHAL_SchedOTAwake_flg : Outport  Port=22
  VHAL_SmartEcoModeSW_flg : Outport  Port=23
  VHAL_UpdCountdownCancel_flg : Outport  Port=24
  VHAL_UpdCountdownSkip_flg : Outport  Port=25
  VHAL_VehACModReq_enum : Outport  Port=26
  wires:
  DT_CAN2_SG_IVI1/1 -> [DT_CAN2_SG_IVI1]
  [DT_CAN2_SG_IVI1] -> bus_selector/1
  bus_selector/1 -> AmbLightColorSet/1(AmbLightColorSet)  "<CAN2_AmbLightColorSet>"
  AmbLightColorSet/1(VHAL_AmbLightColorSet_enum) -> VHAL_AmbLightColorSet_enum/1
  [DT_CAN2_SG_IVI1] -> bus_selector1/1
  bus_selector1/1 -> AmbLightUserSet/1(AmbLightUserSet)  "<CAN2_AmbLightUserSet>"
  AmbLightUserSet/1(VHAL_AmbLightUserSet_enum) -> VHAL_AmbLightUserSet_enum/1
  [DT_CAN2_SG_IVI1] -> bus_selector2/1
  bus_selector2/1 -> BrkAbnGoReadySW/1(BrkAbn_GoReady_SW)  "<CAN2_BrkAbn_GoReady_SW>"
  BrkAbnGoReadySW/1(VHAL_BrkAbnGoReadySW_flg) -> VHAL_BrkAbnGoReadySW_flg/1
  [DT_CAN2_SG_IVI1] -> bus_selector3/1
  bus_selector3/1 -> DRAmbLightBrightnessSet/1(DRAmbLightBrightnessSet)  "<CAN2_DRAmbLightBrightnessSet>"
  DRAmbLightBrightnessSet/1(VHAL_DRAmbLightBrightnessSet_pct) -> VHAL_DRAmbLightBrightnessSet_pct/1
  [DT_CAN2_SG_IVI1] -> bus_selector4/1
  bus_selector4/1 -> FCPFrEvtBtnACMaxReq/1(FCP_FrEvt_BtnACMaxReq)  "<CAN2_FCP_FrEvt_BtnACMaxReq>"
  FCPFrEvtBtnACMaxReq/1(VHAL_FCPFrEvtBtnACMaxReq_flg) -> VHAL_FCPFrEvtBtnACMaxReq_flg/1
  [DT_CAN2_SG_IVI1] -> bus_selector5/1
  bus_selector5/1 -> FCPFrEvtBtnACReq/1(FCP_FrEvt_BtnACReq)  "<CAN2_FCP_FrEvt_BtnACReq>"
  FCPFrEvtBtnACReq/1(VHAL_FCPFrEvtBtnACReq_flg) -> VHAL_FCPFrEvtBtnACReq_flg/1
  [DT_CAN2_SG_IVI1] -> bus_selector6/1
  bus_selector6/1 -> FCPFrEvtBtnAutoReq/1(FCP_FrEvt_BtnAutoReq)  "<CAN2_FCP_FrEvt_BtnAutoReq>"
  FCPFrEvtBtnAutoReq/1(VHAL_FCPFrEvtBtnAutoReq_flg) -> VHAL_FCPFrEvtBtnAutoReq_flg/1
  [DT_CAN2_SG_IVI1] -> bus_selector7/1
  bus_selector7/1 -> FCPFrEvtBtnSyncReq/1(FCP_FrEvt_BtnSyncReq)  "<CAN2_FCP_FrEvt_BtnSyncReq>"
  FCPFrEvtBtnSyncReq/1(VHAL_FCPFrEvtBtnSyncReq_flg) -> VHAL_FCPFrEvtBtnSyncReq_flg/1
  [DT_CAN2_SG_IVI1] -> bus_selector8/1
  bus_selector8/1 -> FCPMidEvtBtnAutoReq/1(FCP_MidEvt_BtnAutoReq)  "<CAN2_FCP_MidEvt_BtnAutoReq>"
  FCPMidEvtBtnAutoReq/1(VHAL_FCPMidEvtBtnAutoReq_flg) -> VHAL_FCPMidEvtBtnAutoReq_flg/1
  [DT_CAN2_SG_IVI1] -> bus_selector9/1
  bus_selector9/1 -> IPAmbLightBrightnessSet/1(IPAmbLightBrightnessSet)  "<CAN2_IPAmbLightBrightnessSet>"
  IPAmbLightBrightnessSet/1(VHAL_IPAmbLightBrightnessSet_pct) -> VHAL_IPAmbLightBrightnessSet_pct/1
  [DT_CAN2_SG_IVI1] -> bus_selector10/1
  bus_selector10/1 -> IVILockSoundSWSta/1(IVI_Lock_SoundSW_Sta)  "<CAN2_IVI_Lock_SoundSW_Sta>"
  IVILockSoundSWSta/1(VHAL_IVILockSoundSWSta_flg) -> VHAL_IVILockSoundSWSta_flg/1
  [DT_CAN2_SG_IVI1] -> bus_selector11/1
  bus_selector11/1 -> IVIOTAUpdSta/1(IVI_OTA_Upd_Sta)  "<CAN2_IVI_OTA_Upd_Sta>"
  IVIOTAUpdSta/1(VHAL_IVIOTAUpdSta_enum) -> VHAL_IVIOTAUpdSta_enum/1
  [DT_CAN2_SG_IVI1] -> bus_selector12/1
  bus_selector12/1 -> LINKtoDrive/1(LINKtoDrive)  "<CAN2_LINKtoDrive>"
  LINKtoDrive/1(VHAL_LINKtoDrive_flg) -> VHAL_LINKtoDrive_flg/1
  [DT_CAN2_SG_IVI1] -> bus_selector13/1
  bus_selector13/1 -> OTACancelDLReq/1(OTA_CancelDL_Req)  "<CAN2_OTA_CancelDL_Req>"
  OTACancelDLReq/1(VHAL_OTACancelDLReq_flg) -> VHAL_OTACancelDLReq_flg/1
  [DT_CAN2_SG_IVI1] -> bus_selector14/1
  bus_selector14/1 -> OTACompNTFYPres/1(OTA_CompNTFY_Pres)  "<CAN2_OTA_CompNTFY_Pres>"
  OTACompNTFYPres/1(VHAL_OTACompNTFYPres_flg) -> VHAL_OTACompNTFYPres_flg/1
  [DT_CAN2_SG_IVI1] -> bus_selector15/1
  bus_selector15/1 -> OTADLReq/1(OTA_DL_Req)  "<CAN2_OTA_DL_Req>"
  OTADLReq/1(VHAL_OTADLReq_flg) -> VHAL_OTADLReq_flg/1
  [DT_CAN2_SG_IVI1] -> bus_selector16/1
  bus_selector16/1 -> OTASuspendDLReq/1(OTA_SuspendDL_Req)  "<CAN2_OTA_SuspendDL_Req>"
  OTASuspendDLReq/1(VHAL_OTASuspendDLReq_flg) -> VHAL_OTASuspendDLReq_flg/1
  [DT_CAN2_SG_IVI1] -> bus_selector17/1
  bus_selector17/1 -> OTAUpdStartReq/1(OTA_UpdStart_Req)  "<CAN2_OTA_UpdStart_Req>"
  OTAUpdStartReq/1(VHAL_OTAUpdStartReq_flg) -> VHAL_OTAUpdStartReq_flg/1
  [DT_CAN2_SG_IVI1] -> bus_selector18/1
  bus_selector18/1 -> OpenDrOpenWdoSW/1(OpenDrOpenWdo_SW)  "<CAN2_OpenDrOpenWdo_SW>"
  OpenDrOpenWdoSW/1(VHAL_OpenDrOpenWdoSW_flg) -> VHAL_OpenDrOpenWdoSW_flg/1
  [DT_CAN2_SG_IVI1] -> bus_selector19/1
  bus_selector19/1 -> PWCLOSEIMD/1(PW_CLOSE_IMD)  "<CAN2_PW_CLOSE_IMD>"
  PWCLOSEIMD/1(VHAL_PWCLOSEIMD_flg) -> VHAL_PWCLOSEIMD_flg/1
  [DT_CAN2_SG_IVI1] -> bus_selector20/1
  bus_selector20/1 -> PWCONTINUEUSE/1(PW_CONTINUE_USE)  "<CAN2_PW_CONTINUE_USE>"
  PWCONTINUEUSE/1(VHAL_PWCONTINUEUSE_flg) -> VHAL_PWCONTINUEUSE_flg/1
  [DT_CAN2_SG_IVI1] -> bus_selector21/1
  bus_selector21/1 -> SchedOTAwake/1(Sched_OTA_wake)  "<CAN2_Sched_OTA_wake>"
  SchedOTAwake/1(VHAL_SchedOTAwake_flg) -> VHAL_SchedOTAwake_flg/1
  [DT_CAN2_SG_IVI1] -> bus_selector22/1
  bus_selector22/1 -> SmartEcoModeSW/1(SmartEco_Mode_SW)  "<CAN2_SmartEco_Mode_SW>"
  SmartEcoModeSW/1(VHAL_SmartEcoModeSW_flg) -> VHAL_SmartEcoModeSW_flg/1
  [DT_CAN2_SG_IVI1] -> bus_selector23/1
  bus_selector23/1 -> UpdCountdownCancel/1(Upd_Countdown_Cancel)  "<CAN2_Upd_Countdown_Cancel>"
  UpdCountdownCancel/1(VHAL_UpdCountdownCancel_flg) -> VHAL_UpdCountdownCancel_flg/1
  [DT_CAN2_SG_IVI1] -> bus_selector24/1
  bus_selector24/1 -> UpdCountdownSkip/1(Upd_Countdown_Skip)  "<CAN2_Upd_Countdown_Skip>"
  UpdCountdownSkip/1(VHAL_UpdCountdownSkip_flg) -> VHAL_UpdCountdownSkip_flg/1
  [DT_CAN2_SG_IVI1] -> bus_selector25/1
  bus_selector25/1 -> VehACModReq/1(VehACModReq)  "<CAN2_VehACModReq>"
  VehACModReq/1(VHAL_VehACModReq_enum) -> VHAL_VehACModReq_enum/1
